simulink model "path_tracking"  (R2024b)
settings: Solver=VariableStepAuto  StartTime=0.0  StopTime=10.0  FixedStep=T  RelTol=1e-3
settings Model: DataDictionary=wrapper2.sldd  Creator=maciej  LastModifiedBy=maciej

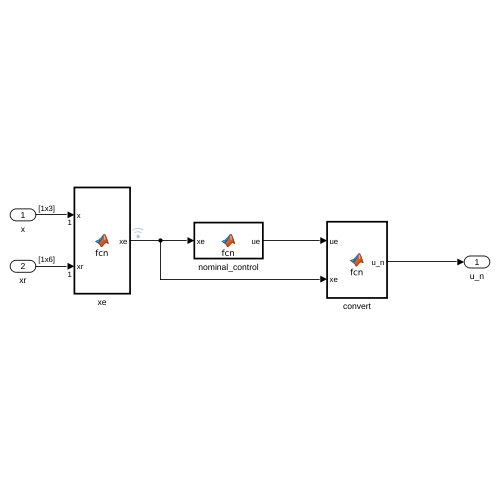
[thumbnail: Simulink's stored preview of the top-level diagram]
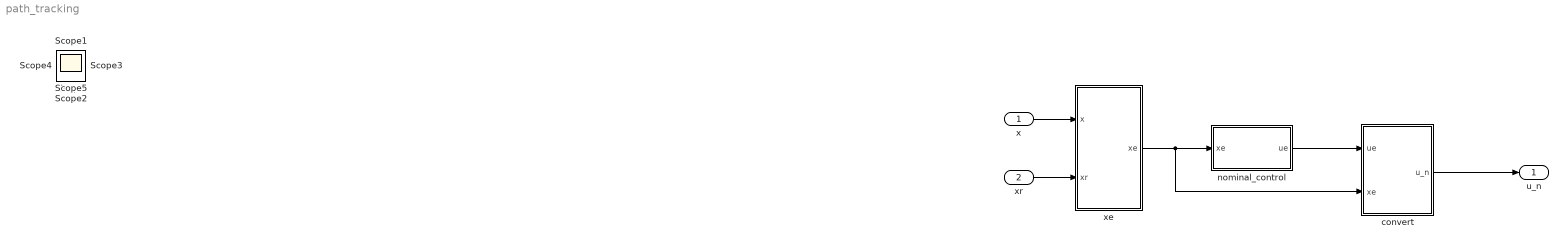
== system path_tracking ==
  x : Inport  PortDimensions=[1 3]
  xr : Inport  Port=2  PortDimensions=[1 6]
  convert : MATLAB Function  TreatAsAtomicUnit=on
  nominal_control : MATLAB Function  TreatAsAtomicUnit=on
  xe : MATLAB Function  TreatAsAtomicUnit=on
  u_n : Outport
  Scope{,1..5} (6 alike) : Scope
  wires:
  nominal_control/1(ue) -> convert/1(ue)
  xr/1 -> xe/2(xr)
  x/1 -> xe/1(x)
  convert/1(u_n) -> u_n/1
  xe/1(xe) -> convert/2(xe), nominal_control/1(xe)

== matlab function path_tracking/xe ==
  data: x input; xe output; xr input
function xe = fcn(x, xr)
    c = cos(x(3));
    s = sin(x(3));
    dx = [xr(1) - x(1); xr(3) - x(2); xr(5) - x(3)];

    xe = [c s 0; -s c 0; 0 0 1] * dx;
end

== matlab function path_tracking/convert ==
  data: ue input; u_n output; xe input
function u_n = fcn(ue, xe)
    v  = cos(xe(3)) - ue(1);
    w = 0 - ue(2);

    u_n = [v, w]';
end

== matlab function path_tracking/nominal_control ==
  data: xe input; ue output
function ue = fcn(xe)
    K = ...
    [ ...
        0.1    0.0000    0.0000; ...
        0.0000   0.1     13.0995 ...
    ];

    ue = -K*xe;
end
